simulink model "MatlabFunction_TestGen_diff11"  (R2017b)
settings: Solver=FixedStepDiscrete  StartTime=0.0  StopTime=10.0  RelTol=1e-3
settings Model: Creator=ktrinh  LastModifiedBy=ktrinh
settings DebuggingCC: ParameterOverflowMsg=none

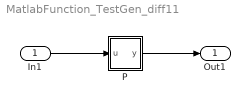
== system MatlabFunction_TestGen_diff11 ==
  In1 : Inport  OutDataTypeStr=single  PortDimensions=[3,3]
  P : MATLAB Function  TreatAsAtomicUnit=on
  Out1 : Outport
  wires:
  In1/1 -> P/1(u)
  P/1(y) -> Out1/1

== matlab function MatlabFunction_TestGen_diff11/P ==
  data: u input; y output
function y = fcn(u)
y = diff(u, 3);
